simulink model "ipsSystem"  (R2018a)
settings: Solver=VariableStepAuto  StartTime=0.0  StopTime=inf  RelTol=1e-3
undefined symbols (not defined in the file): Ion, Lithium
libraries: powerlib x39, electricdrivelib x1, powerlib_meascontrol x1
settings Model: Creator=Rafid  LastModifiedBy=Rafid
settings SolverCC: ZeroCrossAlgorithm=Adaptive
settings DebuggingCC: MaxConsecutiveZCsMsg=none

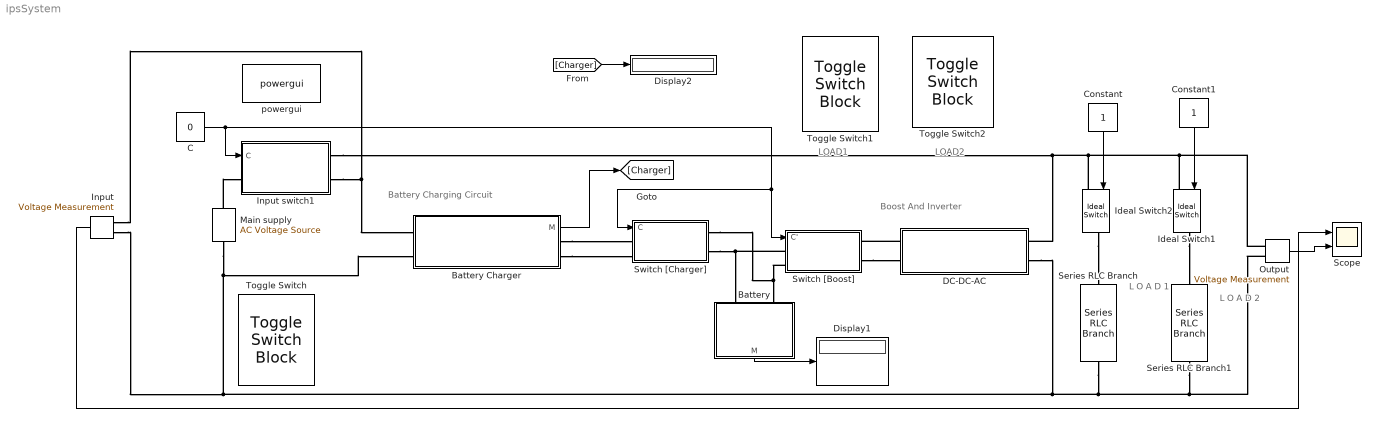
== system ipsSystem ==
  note: L
      | O
      | A
      | D
      | 1
  note: Battery Charging Circuit
  note: Boost And Inverter
  note: L
      | O
      | A
      | D
      | 2
  note: LOAD1
  note: LOAD2
  Battery : Subsystem
  Battery Charger : Subsystem
  C : Constant  Value=0
  Constant : Constant
  Constant1 : Constant
  DC-DC-AC : Subsystem
  Display1 : Display
  Display2 : Display
  Ideal Switch1 : powerlib/Power Electronics/Ideal Switch  Ron=0.001  Lon=0  IC=0  Rs=inf  Cs=inf  Measurements=off
  Ideal Switch2 : powerlib/Power Electronics/Ideal Switch  Ron=0.001  Lon=0  IC=0  Rs=inf  Cs=inf  Measurements=off
  Input : powerlib/Measurements/Voltage Measurement  PhasorSimulation=off  OutputType=Complex  PSBequivalent=0
  Input switch1 : Subsystem
  Main supply : powerlib/Electrical Sources/AC Voltage Source  Amplitude=250  Phase=0  Frequency=50  SampleTime=1/10000  Measurements=None  BusType=swing  Pref=10e3  Qref=0  Qmin=-inf  Qmax=+inf
  Output : powerlib/Measurements/Voltage Measurement  PhasorSimulation=off  OutputType=Complex  PSBequivalent=0
  Scope : Scope  NumInputPorts=2
  Series RLC Branch : powerlib/Elements/Series RLC Branch  LConnTagsString=__new0  RConnTagsString=__new0  BranchType=R  Resistance=10000  Inductance=1e-3  SetiL0=off  InitialCurrent=0  Capacitance=1e-6  Setx0=off  InitialVoltage=0  Measurements=None
  Series RLC Branch1 : powerlib/Elements/Series RLC Branch  LConnTagsString=__new0  RConnTagsString=__new0  BranchType=R  Resistance=10000  Inductance=1e-3  SetiL0=off  InitialCurrent=0  Capacitance=1e-6  Setx0=off  InitialVoltage=0  Measurements=None
  Switch [Boost] : Subsystem
  Switch [Charger] : Subsystem
  Toggle Switch : ToggleSwitchBlock  WebBlockId=224  LabelPosition=Hide
      settings: Values={{'Off', 'On'}, [0 1]}
  Toggle Switch1 : ToggleSwitchBlock  WebBlockId=309  LabelPosition=Hide
      settings: Values={{'Off', 'On'}, [0 1]}
  Toggle Switch2 : ToggleSwitchBlock  WebBlockId=311  LabelPosition=Hide
      settings: Values={{'Off', 'On'}, [0 1]}
  powergui : powerlib/powergui  Priority=1  SimulationMode=Continuous  SampleTime=50e-6  frequency=60  Iterations=50  frequencyindice=0  Pbase=100e6  ErrMax=1e-4  UnitsV=kV  UnitsW=MW  buscounter=0  FunctionMessages=off  echomessages=off  EnableUseOfTLC=off  CurrentSourceSwitches=off  DisableSnubberDevices=off  DisableRonSwitches=off  DisableVfSwitches=off  DisplayEquations=off  SolverType=Tustin/Backward Euler (TBE)  Interpol=off  ExternalGateDelay=off  methode=off  Ts=100  x0status=blocks  SPID=on  SwTol=0  HookPort=off  RestoreLinks=warning  ResistiveCurrentMeasurement=off  Frange=[0:2:500]  Ylog=off  Xlog=on  ShowGrid=off  save=off  variable=ZData  structure=0  ZoomFFT=off  StartTime=0.0  cycles=1  DisplayStyle=1  fundamental=60  FreqAxis=off  MaxFrequency=1000  frequencyindicesteady=1  RmsSteady=1  display=off
  wires:
  [Charger] -> Display2/1
  Battery Charger/1(M) -> [Charger]
  Battery/1(M) -> Display1/1
  C/1 -> Switch [Charger]/1(C), Switch [Boost]/1(C'), Input switch1/1(C)
  Constant/1 -> Ideal Switch2/1
  Constant1/1 -> Ideal Switch1/1
  Output/1 -> Scope/2
  Input/1 -> Scope/1
  connections:
  Output/LConn1 -- Ideal Switch1/LConn1 -- Ideal Switch2/LConn1 -- Input switch1/RConn1 -- DC-DC-AC/RConn1
  Main supply/LConn1 -- Input/LConn2 -- DC-DC-AC/RConn2 -- Series RLC Branch1/RConn1 -- Output/LConn2 -- Series RLC Branch/RConn1 -- Battery Charger/LConn2
  Switch [Boost]/LConn2 -- Switch [Charger]/RConn1 -- Battery/LConn2
  Switch [Boost]/LConn1 -- Battery/LConn1 -- Switch [Charger]/RConn2
  DC-DC-AC/LConn1 -- Switch [Boost]/RConn1
  Switch [Boost]/RConn2 -- DC-DC-AC/LConn2
  Battery Charger/RConn1 -- Switch [Charger]/LConn1
  Battery Charger/RConn2 -- Switch [Charger]/LConn2
  Main supply/RConn1 -- Input switch1/LConn1
  Input switch1/RConn2 -- Battery Charger/LConn1 -- Input/LConn1
  Ideal Switch2/RConn1 -- Series RLC Branch/LConn1
  Ideal Switch1/RConn1 -- Series RLC Branch1/LConn1

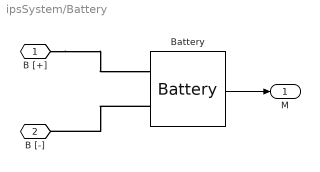
== system ipsSystem/Battery ==
  Battery : electricdrivelib/Extra Sources/Battery  BatType=Lithium-Ion  ShowTempParam=off  ThermalPreset=no  ShowAgeParam=off  NomV=17  NomQ=25.4  SOC=85  Batt_Tr=30  PresetModel=off  MaxQ=25.4  MinV=12  FullV=17.1  Dis_rate=2.3478  R=0.00013333  Normal_OP=24.8835  expZone="[17.05      0.2653]"  current=[6.5 13 32.5]  Units=Time  Tci=20  NomT=20  T2=-30  MaxQ2=4.8  FullV2=7.1  Normal_OP2=5.655  expZone2="[6.58           1]"  Rca=0.6  ti=2000  Dp=0  Neq0=0  Tsim=1e6  Ta1=25  Qeol=5.4*0.9  Reol=0.013333*1.2  Char_age=[2.3478, 3]  Dis_age=[2.3478, 10]  N1=1500  N2=10500  N3=1000  N4=1400  Ta2=45  N5=950
  B [+] : PMIOPort  Side=Left
  B [-] : PMIOPort  Port=2  Side=Left
  M : Outport
  wires:
  Battery/1 -> M/1
  connections:
  Battery/LConn2 -- B [-]/RConn1
  B [+]/RConn1 -- Battery/LConn1

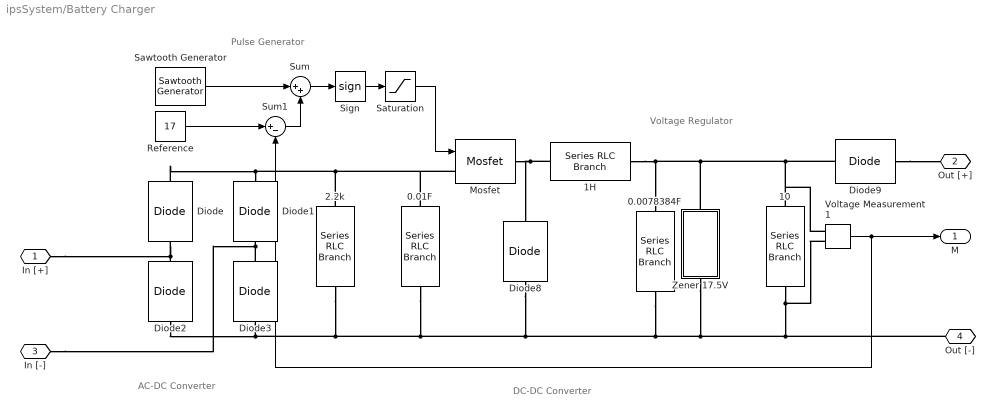
== system ipsSystem/Battery Charger ==
  note: AC-DC Converter
  note: DC-DC Converter
  note: Voltage Regulator
  note: Pulse Generator
  0.0078384F : powerlib/Elements/Series RLC Branch  LConnTagsString=__new0  RConnTagsString=__new0  BranchType=C  Resistance=22  Inductance=1e-3  SetiL0=off  InitialCurrent=0  Capacitance=7.8384e-3  Setx0=off  InitialVoltage=0  Measurements=None
  0.01F : powerlib/Elements/Series RLC Branch  LConnTagsString=__new0  RConnTagsString=__new0  BranchType=C  Resistance=22  Inductance=1e-3  SetiL0=off  InitialCurrent=0  Capacitance=0.01  Setx0=off  InitialVoltage=0  Measurements=None
  10 : powerlib/Elements/Series RLC Branch  LConnTagsString=__new0  RConnTagsString=__new0  BranchType=R  Resistance=10  Inductance=1e-3  SetiL0=off  InitialCurrent=0  Capacitance=1e-6  Setx0=off  InitialVoltage=0  Measurements=None
  1H : powerlib/Elements/Series RLC Branch  LConnTagsString=__new0  RConnTagsString=__new0  BranchType=L  Resistance=22  Inductance=1  SetiL0=off  InitialCurrent=0  Capacitance=1e-6  Setx0=off  InitialVoltage=0  Measurements=None
  2.2k : powerlib/Elements/Series RLC Branch  LConnTagsString=__new0  RConnTagsString=__new0  BranchType=R  Resistance=2200  Inductance=1e-3  SetiL0=off  InitialCurrent=0  Capacitance=1e-6  Setx0=off  InitialVoltage=0  Measurements=None
  Diode{,1..3,8} (5 alike) : powerlib/Power Electronics/Diode  Ron=0.001  Lon=0  Vf=0.8  IC=0  UseSnubber=0  Rs=inf  Cs=inf  Measurements=off
  Diode9 : powerlib/Power Electronics/Diode  Ron=0.001  Lon=0  Vf=0.3  IC=0  UseSnubber=0  Rs=inf  Cs=inf  Measurements=off
  Mosfet : powerlib/Power Electronics/Mosfet  Ron=0.1  Lon=0  Rd=0.01  Vfd=0  IC=0  Rs=inf  Cs=inf  Measurements=off
  Reference : Constant  Value=17
  Saturation : Saturate  UpperLimit=1  LowerLimit=0
  Sawtooth Generator : powerlib_meascontrol/Pulse & Signal Generators/Sawtooth Generator  Freq=50  Phase=180  Ts=0
      settings: SourceProductName=Simscape Power Systems
  Sign : Signum
  Sum : Sum  Inputs=|++
  Sum1 : Sum  Inputs=|+-
  Voltage Measurement1 : powerlib/Measurements/Voltage Measurement  PhasorSimulation=off  OutputType=Complex  PSBequivalent=0
  Zener 17.5V : Subsystem
  In [+] : PMIOPort  Side=Left
  Out [+] : PMIOPort  Port=2  Side=Right
  In [-] : PMIOPort  Port=3  Side=Left
  Out [-] : PMIOPort  Port=4  Side=Right
  M : Outport
  wires:
  Saturation/1 -> Mosfet/1
  Voltage Measurement1/1 -> M/1, Sum1/2
  Sum1/1 -> Sum/2
  Sum/1 -> Sign/1
  Sign/1 -> Saturation/1
  Reference/1 -> Sum1/1
  Sawtooth Generator/1 -> Sum/1
  connections:
  1H/RConn1 -- Diode9/LConn1 -- Voltage Measurement1/LConn1 -- 10/LConn1 -- Zener 17.5V/LConn1 -- 0.0078384F/LConn1
  Diode2/RConn1 -- In [+]/RConn1 -- Diode/LConn1
  Diode3/RConn1 -- In [-]/RConn1 -- Diode1/LConn1
  Voltage Measurement1/LConn2 -- Out [-]/RConn1 -- 0.01F/RConn1 -- Diode2/LConn1 -- Diode3/LConn1 -- 2.2k/RConn1 -- Diode8/LConn1 -- 0.0078384F/RConn1 -- Zener 17.5V/RConn1 -- 10/RConn1
  Diode9/RConn1 -- Out [+]/RConn1
  Mosfet/RConn1 -- Diode8/RConn1 -- 1H/LConn1
  Diode/RConn1 -- Mosfet/LConn1 -- 0.01F/LConn1 -- 2.2k/LConn1 -- Diode1/RConn1

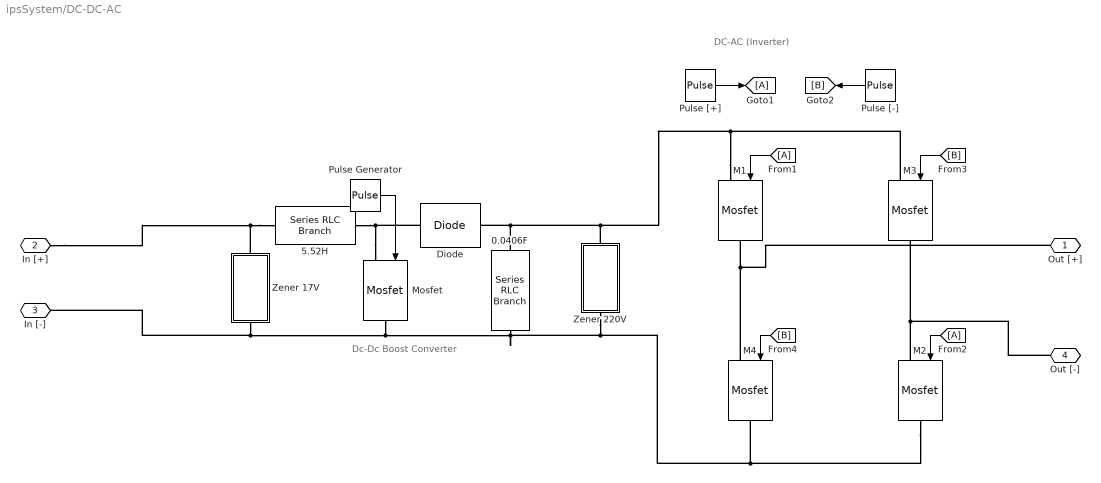
== system ipsSystem/DC-DC-AC ==
  note: Dc-Dc Boost Converter
  note: DC-AC (Inverter)
  0.0406F : powerlib/Elements/Series RLC Branch  LConnTagsString=__new0  RConnTagsString=__new0  BranchType=C  Resistance=1  Inductance=5.513e-2  SetiL0=off  InitialCurrent=0  Capacitance=0.0406  Setx0=off  InitialVoltage=0  Measurements=None
  5.52H : powerlib/Elements/Series RLC Branch  LConnTagsString=__new0  RConnTagsString=__new0  BranchType=L  Resistance=1  Inductance=5.525  SetiL0=off  InitialCurrent=0  Capacitance=1e-6  Setx0=off  InitialVoltage=0  Measurements=None
  Diode : powerlib/Power Electronics/Diode  Ron=0.001  Lon=0  Vf=0.8  IC=0  UseSnubber=0  Rs=inf  Cs=inf  Measurements=off
  M{1..4} (4 alike) : powerlib/Power Electronics/Mosfet  Ron=0.1  Lon=0  Rd=0.01  Vfd=0  IC=0  Rs=1e5  Cs=inf  Measurements=off
  Mosfet : powerlib/Power Electronics/Mosfet  Ron=0.1  Lon=0  Rd=0.01  Vfd=0  IC=0  Rs=1e5  Cs=inf  Measurements=off
  Pulse Generator : DiscretePulseGenerator  PulseType=Time based  Period=0.02  PulseWidth=92.5
  Pulse [+] : DiscretePulseGenerator  PulseType=Time based  Period=0.02  PulseWidth=50
  Pulse [-] : DiscretePulseGenerator  PulseType=Time based  Period=0.02  PulseWidth=50  PhaseDelay=0.01
  Zener 17V : Subsystem
  Zener 220V : Subsystem
  Out [+] : PMIOPort  Side=Right
  In [+] : PMIOPort  Port=2  Side=Left
  In [-] : PMIOPort  Port=3  Side=Left
  Out [-] : PMIOPort  Port=4  Side=Right
  wires:
  [A] -> M1/1
  [B] -> M3/1
  [B] -> M4/1
  Pulse [-]/1 -> [B]
  Pulse [+]/1 -> [A]
  [A] -> M2/1
  Pulse Generator/1 -> Mosfet/1
  connections:
  M2/RConn1 -- M4/RConn1 -- In [-]/RConn1 -- Zener 17V/RConn1 -- Mosfet/RConn1 -- 0.0406F/RConn1 -- Zener 220V/RConn1
  M2/LConn1 -- Out [-]/RConn1 -- M3/RConn1
  M1/LConn1 -- Zener 220V/LConn1 -- 0.0406F/LConn1 -- Diode/RConn1 -- M3/LConn1
  M4/LConn1 -- Out [+]/RConn1 -- M1/RConn1
  Mosfet/LConn1 -- Diode/LConn1 -- 5.52H/RConn1
  5.52H/LConn1 -- In [+]/RConn1 -- Zener 17V/LConn1

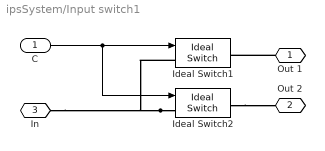
== system ipsSystem/Input switch1 ==
  C : Inport
  Ideal Switch1 : powerlib/Power Electronics/Ideal Switch  Ron=0.001  Lon=0  IC=0  Rs=inf  Cs=inf  Measurements=off
  Ideal Switch2 : powerlib/Power Electronics/Ideal Switch  Ron=0.001  Lon=0  IC=0  Rs=inf  Cs=inf  Measurements=off
  Out 1 : PMIOPort  Side=Right
  Out 2 : PMIOPort  Port=2  Side=Right
  In : PMIOPort  Port=3  Side=Left
  wires:
  C/1 -> Ideal Switch1/1, Ideal Switch2/1
  connections:
  Out 1/RConn1 -- Ideal Switch1/RConn1
  Ideal Switch2/LConn1 -- Ideal Switch1/LConn1 -- In/RConn1
  Ideal Switch2/RConn1 -- Out 2/RConn1

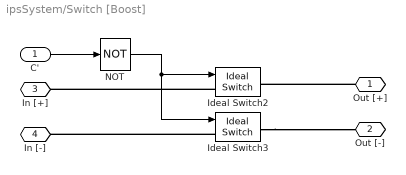
== system ipsSystem/Switch [Boost] ==
  C' : Inport
  Ideal Switch2 : powerlib/Power Electronics/Ideal Switch  Ron=0.001  Lon=0  IC=0  Rs=inf  Cs=inf  Measurements=off
  Ideal Switch3 : powerlib/Power Electronics/Ideal Switch  Ron=0.001  Lon=0  IC=0  Rs=inf  Cs=inf  Measurements=off
  NOT : Logic  Operator=NOT  IconShape=distinctive  AllPortsSameDT=off  OutDataTypeStr=boolean
  Out [+] : PMIOPort  Side=Right
  Out [-] : PMIOPort  Port=2  Side=Right
  In [+] : PMIOPort  Port=3  Side=Left
  In [-] : PMIOPort  Port=4  Side=Left
  wires:
  C'/1 -> NOT/1
  NOT/1 -> Ideal Switch2/1, Ideal Switch3/1
  connections:
  Ideal Switch2/LConn1 -- In [+]/RConn1
  Out [+]/RConn1 -- Ideal Switch2/RConn1
  Ideal Switch3/RConn1 -- Out [-]/RConn1
  Ideal Switch3/LConn1 -- In [-]/RConn1

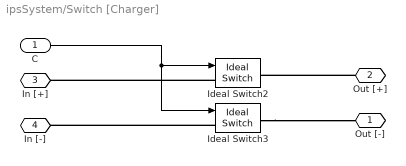
== system ipsSystem/Switch [Charger] ==
  C : Inport
  Ideal Switch2 : powerlib/Power Electronics/Ideal Switch  Ron=0.001  Lon=0  IC=0  Rs=inf  Cs=inf  Measurements=off
  Ideal Switch3 : powerlib/Power Electronics/Ideal Switch  Ron=0.001  Lon=0  IC=0  Rs=inf  Cs=inf  Measurements=off
  Out [-] : PMIOPort  Side=Right
  Out [+] : PMIOPort  Port=2  Side=Right
  In [+] : PMIOPort  Port=3  Side=Left
  In [-] : PMIOPort  Port=4  Side=Left
  wires:
  C/1 -> Ideal Switch2/1, Ideal Switch3/1
  connections:
  Ideal Switch2/LConn1 -- In [+]/RConn1
  Out [+]/RConn1 -- Ideal Switch2/RConn1
  Ideal Switch3/RConn1 -- Out [-]/RConn1
  Ideal Switch3/LConn1 -- In [-]/RConn1

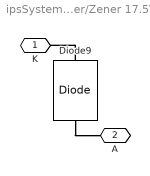
== system ipsSystem/Battery Charger/Zener 17.5V ==
  Diode9 : powerlib/Power Electronics/Diode  Ron=0.001  Lon=0  Vf=17.5  IC=0  UseSnubber=0  Rs=inf  Cs=inf  Measurements=off
  K : PMIOPort  Side=Left
  A : PMIOPort  Port=2  Side=Right
  connections:
  Diode9/RConn1 -- A/RConn1
  Diode9/LConn1 -- K/RConn1

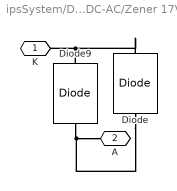
== system ipsSystem/DC-DC-AC/Zener 17V ==
  Diode : powerlib/Power Electronics/Diode  Ron=0.001  Lon=0  Vf=0.8  IC=0  UseSnubber=0  Rs=inf  Cs=inf  Measurements=off
  Diode9 : powerlib/Power Electronics/Diode  Ron=0.001  Lon=0  Vf=17  IC=0  UseSnubber=0  Rs=inf  Cs=inf  Measurements=off
  K : PMIOPort  Side=Left
  A : PMIOPort  Port=2  Side=Right
  connections:
  Diode9/RConn1 -- Diode/LConn1 -- A/RConn1
  Diode9/LConn1 -- Diode/RConn1 -- K/RConn1

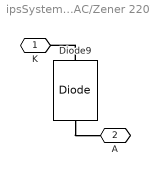
== system ipsSystem/DC-DC-AC/Zener 220V ==
  Diode9 : powerlib/Power Electronics/Diode  Ron=0.001  Lon=0  Vf=220  IC=0  UseSnubber=0  Rs=inf  Cs=inf  Measurements=off
  K : PMIOPort  Side=Left
  A : PMIOPort  Port=2  Side=Right
  connections:
  Diode9/RConn1 -- A/RConn1
  Diode9/LConn1 -- K/RConn1
